simulink model "Subsystem"  (R2020b)
settings: Solver=VariableStepAuto  StartTime=0.0  StopTime=300  RelTol=1e-3
settings Model: DataDictionary=Cruise_data.sldd  Creator=HP  LastModifiedBy=HP
settings DataIOCC: SaveOutput=off  SaveTime=off

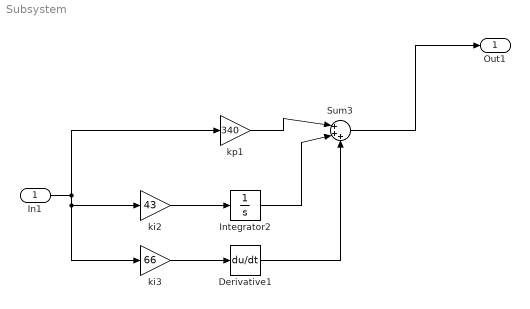
== system Subsystem ==
  In1 : Inport  OutDataTypeStr=double  PortDimensions=1  SampleTime=0
  Derivative1 : Derivative
  Integrator2 : Integrator
  Sum3 : Sum  Inputs=|+++
  ki2 : Gain  Gain=43
  ki3 : Gain  Gain=66
  kp1 : Gain  Gain=340
  Out1 : Outport  OutDataTypeStr=double  PortDimensions=1  SampleTime=0
  wires:
  Sum3/1 -> Out1/1
  ki2/1 -> Integrator2/1
  In1/1 -> kp1/1, ki3/1, ki2/1
  Integrator2/1 -> Sum3/2
  ki3/1 -> Derivative1/1
  kp1/1 -> Sum3/1
  Derivative1/1 -> Sum3/3
